simulink subsystem "motorDPT"  (R2021b)
settings: Solver=VariableStepAuto  StartTime=0.0  StopTime=10.0  RelTol=1e-3
undefined symbols (not defined in the file): J, ke, km, L, R
settings Model: Creator=vital  LastModifiedBy=vital
settings SolverCC: AlgebraicLoopSolver=TrustRegion
settings DebuggingCC: SFMachineParentedDataDiag=warning

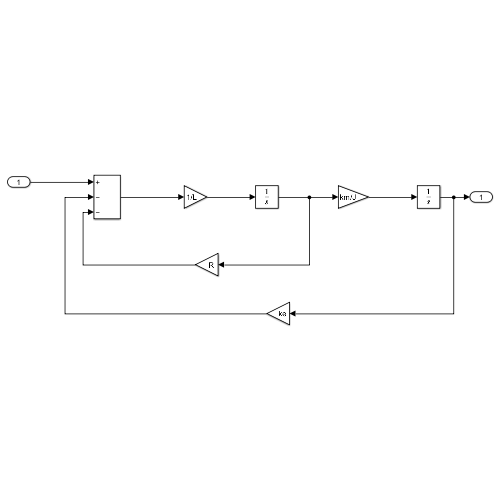
[thumbnail: Simulink's stored preview of the top-level diagram]
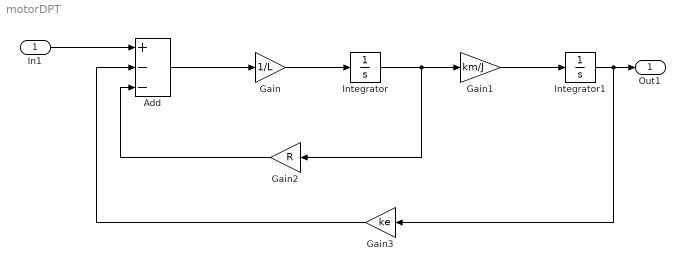
== system motorDPT ==
  In1 : Inport
  Add : Sum  Inputs=+--
  Gain : Gain  Gain=1/L
  Gain1 : Gain  Gain=km/J
  Gain2 : Gain  Gain=R
  Gain3 : Gain  Gain=ke
  Integrator : Integrator
  Integrator1 : Integrator
  Out1 : Outport
  wires:
  Gain3/1 -> Add/2
  Integrator1/1 -> Out1/1, Gain3/1
  Gain1/1 -> Integrator1/1
  Gain2/1 -> Add/3
  Integrator/1 -> Gain1/1, Gain2/1
  Gain/1 -> Integrator/1
  Add/1 -> Gain/1
  In1/1 -> Add/1
